simulink model "pendulum_control"  (Simulink 5.0)
settings: Solver=ode4  StartTime=0.0  StopTime=10.0  FixedStep=0.001  RelTol=1e-3
undefined symbols (not defined in the file): g, l, m, rtai_lib, Scope
settings Model: Creator=attolico  LastModifiedBy=attolico  ExtModeAutoUpdateStatusClock=off  RTWSystemTargetFile=rtai.tlc  RTWTemplateMakefile=rtai.tmf  RTWGenerateCodeOnly=on  RTWOptions="-aEnforceIntegerDowncast=1 -aFoldNonRolledExpr=1 -aForceParamTrailComments=0 -aGenerateComments=1 -aGenerateReport=0 -aIncDataTypeInIds=0 -aIncHierarchyInIds=0 -aInlineInvariantSignals=0 -aInlinedPrmAccess=\"Literals\" -aLocalBlockOutputs=1 -aMaxRTWIdLen=31 -aPrefixModelToSubsysFcnNames=1 -aRTWVerbose=1 -aRollThreshold=5 -aShowEliminatedStatements=0"

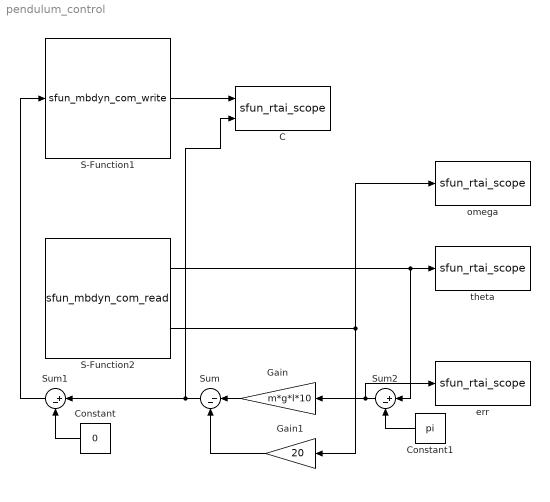
== system pendulum_control ==
  C : S-Function  AncestorBlock=rtai_lib/Scope  FunctionName=sfun_rtai_scope  Parameters=numch,ts  mask(RTAI SCOPE){numch=2, ts=0.001}
      mask prompts: numch "Channels:"; ts "Sampling Time (-1 for inherited)"
      mask help: RTAI run-time scope
      mask StyleString: popup(1|2|3|4|5),edit
  Constant : Constant  Orientation=left  Value=0
  Constant1 : Constant  Orientation=left  Value=pi
  Gain : Gain  Orientation=left  Gain=m*g*l*10  SaturateOnIntegerOverflow=on
  Gain1 : Gain  Orientation=left  Gain=20  SaturateOnIntegerOverflow=on
  S-Function1 : S-Function  FunctionName=sfun_mbdyn_com_write  Parameters='127.0.0.1','mbdtsk','MBXOUT',1,0.001
  S-Function2 : S-Function  FunctionName=sfun_mbdyn_com_read  Parameters='127.0.0.1','mbdtsk','MBXINN',2,0.001
  Sum : Sum  Orientation=left  Inputs=|--  SaturateOnIntegerOverflow=on
  Sum1 : Sum  Orientation=left  Inputs=|+-  SaturateOnIntegerOverflow=on
  Sum2 : Sum  Orientation=left  Inputs=|+-  SaturateOnIntegerOverflow=on
  err : S-Function  AncestorBlock=rtai_lib/Scope  FunctionName=sfun_rtai_scope  Parameters=numch,ts  mask(RTAI SCOPE){numch=1, ts=0.001}
      mask prompts: numch "Channels:"; ts "Sampling Time (-1 for inherited)"
      mask help: RTAI run-time scope
      mask StyleString: popup(1|2|3|4|5),edit
  omega : S-Function  AncestorBlock=rtai_lib/Scope  FunctionName=sfun_rtai_scope  Parameters=numch,ts  mask(RTAI SCOPE){numch=1, ts=0.001}
      mask prompts: numch "Channels:"; ts "Sampling Time (-1 for inherited)"
      mask help: RTAI run-time scope
      mask StyleString: popup(1|2|3|4|5),edit
  theta : S-Function  AncestorBlock=rtai_lib/Scope  FunctionName=sfun_rtai_scope  Parameters=numch,ts  mask(RTAI SCOPE){numch=1, ts=0.001}
      mask prompts: numch "Channels:"; ts "Sampling Time (-1 for inherited)"
      mask help: RTAI run-time scope
      mask StyleString: popup(1|2|3|4|5),edit
  wires:
  S-Function2/1 -> theta/1, Sum2/1
  Gain/1 -> Sum/1
  Gain1/1 -> Sum/2
  Sum/1 -> Sum1/1, C/2
  S-Function1/1 -> C/1
  Sum1/1 -> S-Function1/1
  Constant/1 -> Sum1/2
  Sum2/1 -> Gain/1, err/1
  Constant1/1 -> Sum2/2
  S-Function2/2 -> omega/1, Gain1/1
